simulink model "Battery_iDesignMask"  (R2020b)
settings: Solver=FixedStepAuto  StartTime=0.0  StopTime=10000  FixedStep=0.01  RelTol=1e-3  EnableMultiTasking=on
undefined symbols (not defined in the file or in its folder): Ion, Li
libraries: simulink x4, PB_Library_Master x1, TemperatureBlock x1
settings Model: PauseTimes=184  Creator=ewong  LastModifiedBy=nbutler2
settings DataIOCC: ReturnWorkspaceOutputs=off
settings OptimizationCC: LifeSpan=inf
settings DebuggingCC: PregeneratedLibrarySubsystemCodeDiagnostic=none  SFUnexpectedBacktrackingDiag=warning  SFNoUnconditionalDefaultTransitionDiag=warning  SFExecutionAtInitializationDiag=none  ArithmeticOperatorsInVariantConditions=warning
settings SFSimCC: SimUseLocalCustomCode=off  CustomCodeUndefinedFunction=UseInterfaceOnly
settings RTWCC: RTWUseLocalCustomCode=off
settings CodeAppCC: StateflowObjectComments=on
settings GRTTargetCC: TargetLangStandard=C89/C90 (ANSI)
settings ConfigComp: CovMetricSettings=dw  CovSaveCumulativeToWorkspaceVar=on  CovSaveSingleToWorkspaceVar=on  CovExternalEMLEnable=off

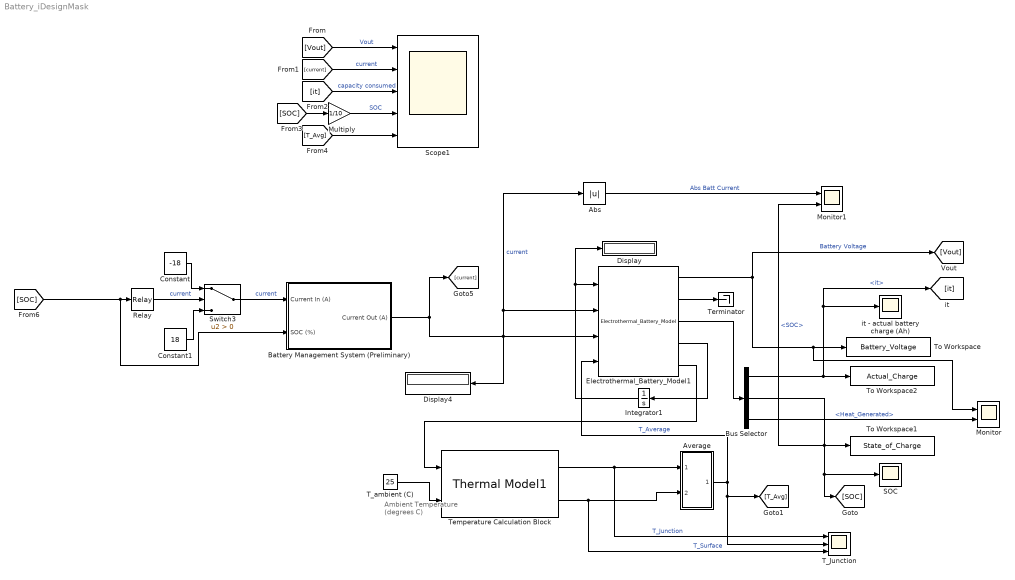
== system Battery_iDesignMask ==
  note: Ambient Temperature
      | (degrees C)
  Abs : Abs
  Average : Subsystem
  Battery Management System (Preliminary) : Subsystem
  Bus Selector : BusSelector  OutputSignals=it,SOC,Heat_Generated
  Constant : Constant  Value=-18
  Constant1 : Constant  Value=18
  Display : Display
  Display4 : Display
  Electrothermal_Battery_Model1 : PB_Library_Master/Electrothermal_Battery_Model  E0_M=E0_M  Q_M=Q_M  R_M=R_M  K_M=K_M  B_M=B_M  SOC_Init_M=SOC_Init_M  A_M=A_M  battery_type_M=Li-Ion  TempIn=Celsius  BWS=on  thermal=on  nameField=Thermal Model
  Integrator1 : Integrator
  Monitor : Scope  NumInputPorts=2
  Monitor1 : Scope  NumInputPorts=2
  Multiply : Gain  Gain=1/10
  Relay : Relay  OnSwitchValue=99  OffSwitchValue=5  OnOutputValue=0  OffOutputValue=1
  SOC : Scope
  Scope1 : Scope  NumInputPorts=5
  Switch3 : Switch  Criteria=u2 > Threshold
  T_Junction : Scope  NumInputPorts=3
  T_ambient (C) : Constant  Value=25
  Temperature Calculation Block : TemperatureBlock/Thermal Model1  Tj_0_M=Tj_0_M  Ts_0_M=Ts_0_M  Cj_M=Cj_M  Rj_M=Rj_M  Cs_M=Cs_M  Ru_M=Ru_M  TempIn=Celsius  TempOut=Celsius
  Terminator : Terminator
  To Workspace : ToWorkspace  VariableName=Battery_Voltage  SampleTime=-1
  To Workspace1 : ToWorkspace  VariableName=State_of_Charge  SampleTime=-1
  To Workspace2 : ToWorkspace  VariableName=Actual_Charge  SampleTime=-1
  it - actual battery charge (Ah) : Scope
  wires:
  Bus Selector/2 -> [SOC], SOC/1, Monitor1/2, To Workspace1/1  "<SOC>"
  Electrothermal_Battery_Model1/1 -> [Vout], Monitor/1, To Workspace/1  "Battery Voltage"
  Bus Selector/1 -> To Workspace2/1, [it], it - actual battery charge (Ah)/1  "<it>"
  Electrothermal_Battery_Model1/3 -> Bus Selector/1
  Electrothermal_Battery_Model1/4 -> Integrator1/1
  Electrothermal_Battery_Model1/2 -> Terminator/1
  Integrator1/1 -> Electrothermal_Battery_Model1/1, Display/1
  T_ambient (C)/1 -> Temperature Calculation Block/2
  Bus Selector/3 -> Monitor/2  "<Heat_Generated>"
  Abs/1 -> Monitor1/1  "Abs Batt Current"
  Electrothermal_Battery_Model1/5 -> Temperature Calculation Block/1
  Temperature Calculation Block/1 -> T_Junction/1, Average/1(In1)  "T_Junction"
  Temperature Calculation Block/2 -> T_Junction/3, Average/2(In2)  "T_Surface"
  Average/1(Out1) -> Electrothermal_Battery_Model1/4, [T_Avg], T_Junction/2  "T_Average"
  Battery Management System (Preliminary)/1(Current Out (A)) -> [current], Electrothermal_Battery_Model1/3, Display4/1, Electrothermal_Battery_Model1/2, Abs/1  "current"
  [SOC] -> Battery Management System (Preliminary)/2(SOC (%)), Relay/1
  Constant1/1 -> Switch3/3
  Constant/1 -> Switch3/1
  Relay/1 -> Switch3/2  "current"
  Switch3/1 -> Battery Management System (Preliminary)/1(Current In (A))  "current"
  [Vout] -> Scope1/1  "Vout"
  [current] -> Scope1/2  "current"
  [it] -> Scope1/3  "capacity consumed"
  [SOC] -> Multiply/1
  Multiply/1 -> Scope1/4  "SOC"
  [T_Avg] -> Scope1/5

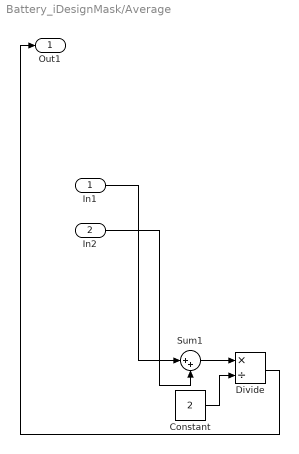
== system Battery_iDesignMask/Average ==
  In1 : Inport
  In2 : Inport  Port=2
  Constant : Constant  Value=2
  Divide : Product  Inputs=*/
  Sum1 : Sum  Inputs=|++
  Out1 : Outport  VectorParamsAs1DForOutWhenUnconnected=off
  wires:
  In1/1 -> Sum1/1
  Sum1/1 -> Divide/1
  In2/1 -> Sum1/2
  Constant/1 -> Divide/2
  Divide/1 -> Out1/1

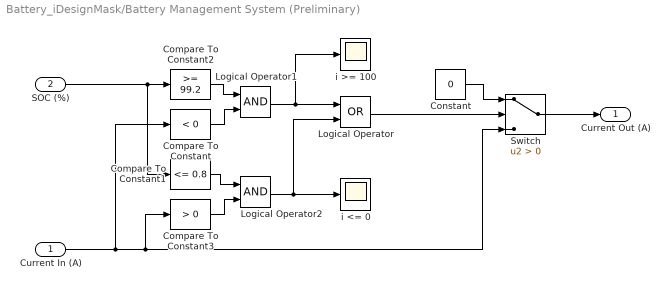
== system Battery_iDesignMask/Battery Management System (Preliminary) ==
  Current In (A) : Inport
  SOC (%) : Inport  Port=2
  Compare To Constant : simulink/Logic and Bit Operations/Compare To Constant  relop=<  const=0  OutDataTypeStr=boolean
  Compare To Constant1 : simulink/Logic and Bit Operations/Compare To Constant  relop=<=  const=0.8  OutDataTypeStr=boolean
  Compare To Constant2 : simulink/Logic and Bit Operations/Compare To Constant  relop=>=  const=99.2  OutDataTypeStr=boolean
  Compare To Constant3 : simulink/Logic and Bit Operations/Compare To Constant  relop=>  const=0  OutDataTypeStr=boolean
  Constant : Constant  Value=0
  Logical Operator : Logic  Operator=OR  AllPortsSameDT=off  OutDataTypeStr=boolean
  Logical Operator1 : Logic  AllPortsSameDT=off  OutDataTypeStr=boolean
  Logical Operator2 : Logic  AllPortsSameDT=off  OutDataTypeStr=boolean
  Switch : Switch  Criteria=u2 > Threshold
  i <= 0 : Scope
  i >= 100 : Scope
  Current Out (A) : Outport  VectorParamsAs1DForOutWhenUnconnected=off
  wires:
  Constant/1 -> Switch/1
  Logical Operator/1 -> Switch/2
  Current In (A)/1 -> Compare To Constant/1, Compare To Constant3/1, Switch/3
  SOC (%)/1 -> Compare To Constant1/1, Compare To Constant2/1
  Compare To Constant2/1 -> Logical Operator1/1
  Compare To Constant/1 -> Logical Operator1/2
  Compare To Constant1/1 -> Logical Operator2/1
  Compare To Constant3/1 -> Logical Operator2/2
  Logical Operator1/1 -> i >= 100/1, Logical Operator/1
  Logical Operator2/1 -> i <= 0/1, Logical Operator/2
  Switch/1 -> Current Out (A)/1
